simulink model "ModelPendulum"  (R2024a)
settings: Solver=VariableStepAuto  StartTime=0.0  StopTime=T_sim  RelTol=1e-3
undefined symbols (not defined in the file or in its folder): model, Ts_ensaio
settings Model: Creator=Douglas  LastModifiedBy=Douglas

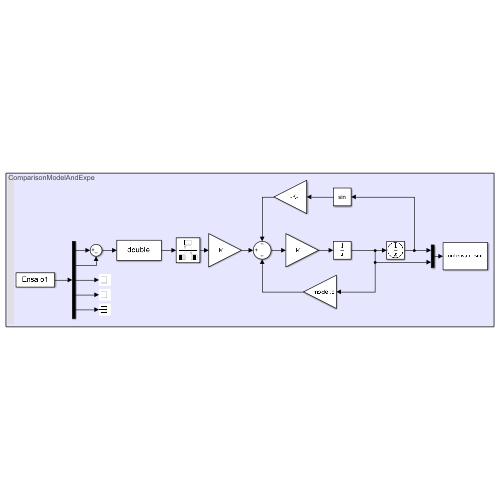
[thumbnail: Simulink's stored preview of the top-level diagram]
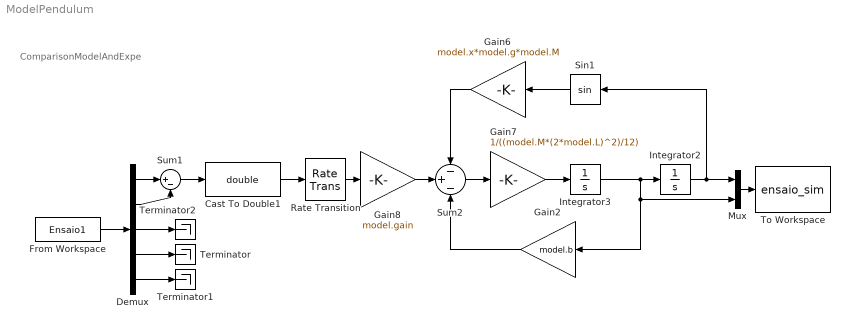
== system ModelPendulum ==
  note: ComparisonModelAndExpe
  Cast To Double1 : DataTypeConversion  OutDataTypeStr=double  SaturateOnIntegerOverflow=off  RndMeth=Floor
  Demux : Demux  Outputs=5
  From Workspace : FromWorkspace  VariableName=Ensaio1  SampleTime=Ts_ensaio
  Gain2 : Gain  Gain=model.b
  Gain6 : Gain  Gain=model.x*model.g*model.M
  Gain7 : Gain  Gain=1/((model.M*(2*model.L)^2)/12)
  Gain8 : Gain  Gain=model.gain
  Integrator2 : Integrator  WrapState=on
  Integrator3 : Integrator
  Mux : Mux  Inputs=2
  Rate Transition : RateTransition
  Sin1 : Trigonometry
  Sum1 : Sum  Inputs=|+-
  Sum2 : Sum  Inputs=-+-
  Terminator : Terminator
  Terminator1 : Terminator
  Terminator2 : Terminator
  To Workspace : ToWorkspace  VariableName=ensaio_sim  SaveFormat=Structure  SampleTime=Ts_ensaio
  wires:
  Cast To Double1/1 -> Rate Transition/1
  Sum1/1 -> Cast To Double1/1
  Gain7/1 -> Integrator3/1
  Integrator3/1 -> Integrator2/1, Gain2/1, Mux/2
  Gain8/1 -> Sum2/2
  Gain6/1 -> Sum2/1
  From Workspace/1 -> Demux/1
  Gain2/1 -> Sum2/3
  Sum2/1 -> Gain7/1
  Sin1/1 -> Gain6/1
  Integrator2/1 -> Mux/1, Sin1/1
  Demux/1 -> Sum1/1
  Demux/2 -> Sum1/2
  Rate Transition/1 -> Gain8/1
  Demux/4 -> Terminator/1
  Demux/5 -> Terminator1/1
  Demux/3 -> Terminator2/1
  Mux/1 -> To Workspace/1
